simulink model "modularPlant_th"  (R2018b)
settings: Solver=ode15s  StartTime=0.0  StopTime=sim_time  MaxStep=5  RelTol=1e-3  AbsTol=1e-3
values from neighbouring files (symbols this model uses):
  elevonDeflection = [0 0]'*pi/180    [ayazPlant_ts.m]    (also in modularPlant_ts.m)
  winchSpeeds = 0.1*[1 1 1]'    [ayazPlant_ts.m]    (also in modularPlant_ts.m)
  windDir = 0    [ayazPlant_ts.m]    (also in modularPlant_ts.m)
  windSpeed = 1.5    [ayazPlant_ts.m]    (also in modularPlant_ts.m)
libraries: modularPlant_cl x1
settings Model: Creator=mcobb  LastModifiedBy=mcobb

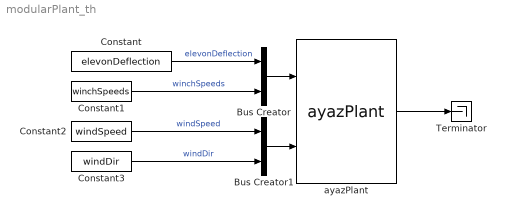
== system modularPlant_th ==
  Bus Creator : BusCreator  Inputs=2
  Bus Creator1 : BusCreator  Inputs=2
  Constant : Constant  Value=elevonDeflection
  Constant1 : Constant  Value=winchSpeeds
  Constant2 : Constant  Value=windSpeed
  Constant3 : Constant  Value=windDir
  Terminator : Terminator
  ayazPlant : modularPlant_cl/ayazPlant  SystemSampleTime=-1
  wires:
  Bus Creator/1 -> ayazPlant/1
  Bus Creator1/1 -> ayazPlant/2
  Constant/1 -> Bus Creator/1  "elevonDeflection"
  Constant1/1 -> Bus Creator/2  "winchSpeeds"
  Constant3/1 -> Bus Creator1/2  "windDir"
  Constant2/1 -> Bus Creator1/1  "windSpeed"
  ayazPlant/1 -> Terminator/1
